simulink model "Prova_inversione"  (R2015a)
settings: Solver=ode45  StartTime=0.0  StopTime=10.0  RelTol=1e-3
values from neighbouring files (symbols this model uses):
  b = 0.55/2    (= 0.275)    [TiltCopter_Parameters.m]
  Kq = Cq*ro*A*R^3    (= 2.88925724261e-07)    [TiltCopter_Parameters.m]
  Kt = Ct*ro*A*R^2    (= 2.46191978476e-05)    [TiltCopter_Parameters.m]
  omega_hover = OMEhov    [TiltCopter_Parameters.m]
settings Model: Creator=Claudio  LastModifiedBy=Claudio

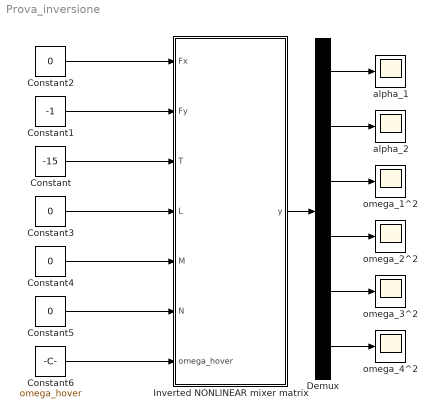
== system Prova_inversione ==
  Constant : Constant  Value=-15
  Constant1 : Constant  Value=-1
  Constant{2..5} (4 alike) : Constant  Value=0
  Constant6 : Constant  Value=omega_hover
  Demux : Demux  Outputs=6
  Inverted NONLINEAR mixer matrix : MATLAB Function  TreatAsAtomicUnit=on
  alpha_1 : Scope
  alpha_2 : Scope
  omega_1^2 : Scope
      settings: SaveName=ScopeData2
  omega_2^2 : Scope
      settings: SaveName=ScopeData3
  omega_3^2 : Scope
      settings: SaveName=ScopeData4
  omega_4^2 : Scope
      settings: SaveName=ScopeData5
  wires:
  Constant/1 -> Inverted NONLINEAR mixer matrix/3(T)
  Constant1/1 -> Inverted NONLINEAR mixer matrix/2(Fy)
  Constant2/1 -> Inverted NONLINEAR mixer matrix/1(Fx)
  Constant3/1 -> Inverted NONLINEAR mixer matrix/4(L)
  Constant4/1 -> Inverted NONLINEAR mixer matrix/5(M)
  Constant5/1 -> Inverted NONLINEAR mixer matrix/6(N)
  Constant6/1 -> Inverted NONLINEAR mixer matrix/7(omega_hover)
  Demux/6 -> omega_4^2/1
  Demux/5 -> omega_3^2/1
  Demux/4 -> omega_2^2/1
  Demux/3 -> omega_1^2/1
  Demux/2 -> alpha_2/1
  Demux/1 -> alpha_1/1
  Inverted NONLINEAR mixer matrix/1(y) -> Demux/1

== matlab function Prova_inversione/Inverted NONLINEAR mixer matrix ==
  data: Fx input; Fy input; T input; L input; M input; N input; y output; omega_hover input; Kt parameter; Kq parameter; b parameter
function y = fcn(Fx,Fy,T,L,M,N,omega_hover,Kt,Kq,b)
%#codegen

omega_1 = omega_hover;
omega_2 = omega_hover;
omega_3 = omega_hover;
omega_4 = omega_hover;

% Calcolo prima gli alpha per ottenere la Fx e Fy desiderata considerando
% una omega di hovering
alpha_2 = -asin(Fx/(Kt*(omega_2^2 + omega_4^2)));

alpha_1 = asin(Fy/(Kt*(omega_1^2 + omega_3^2)));
alpha_3 = -alpha_1;
alpha_4 = -alpha_2;

% A questo punto risolvo la matrice K_mix, considerando gli angoli noti e
% risolvo solo per omega_i
K_mix = [
    -Kt*cos(alpha_1),                      -Kt*cos(alpha_2),                    -Kt*cos(alpha_3),                    -Kt*cos(alpha_4);
                                   0, - Kq*sin(alpha_2) - Kt*b*cos(alpha_2),                                   0, Kq*sin(alpha_4) + Kt*b*cos(alpha_4);
 Kt*b*cos(alpha_1) - Kq*sin(alpha_1),                                     0, Kq*sin(alpha_3) - Kt*b*cos(alpha_3),                                   0;
 Kq*cos(alpha_1) + Kt*b*sin(alpha_1),   Kt*b*sin(alpha_2) - Kq*cos(alpha_2), Kq*cos(alpha_3) + Kt*b*sin(alpha_3), Kt*b*sin(alpha_4) - Kq*cos(alpha_4)]

Omega_result = inv(K_mix)*[T;L;M;N];
y = [alpha_1;alpha_2;Omega_result];
